simulink model "Sim_Riementrieb"  (R2019b)
settings: Solver=ode45  StartTime=0.0  StopTime=12  MaxStep=1e-3  RelTol=1e-7  AbsTol=1e-7  EnableMultiTasking=on
undefined symbols (not defined in the file or in its folder): parSys
libraries: cstblocks x2
settings Model: Creator=wke  LastModifiedBy=GF
settings SolverCC: AutoScaleAbsTol=off  ShapePreserveControl=EnableAll
settings DataIOCC: LimitDataPoints=on  SaveFormat=Array  SignalLoggingSaveFormat=ModelDataLogs  ReturnWorkspaceOutputs=off
settings OptimizationCC: ExpressionDepthLimit=2147483647  LifeSpan=inf
settings DebuggingCC: UnderspecifiedInitializationDetection=Classic  MergeDetectMultiDrivingBlocksExec=none  SolverPrmCheckMsg=warning  FcnCallInpInsideContextMsg=warning  StateNameClashWarn=warning  SFUnexpectedBacktrackingDiag=warning  SFNoUnconditionalDefaultTransitionDiag=warning  SFExecutionAtInitializationDiag=none  ArithmeticOperatorsInVariantConditions=warning
settings HardwareCC: ProdBitPerPointer=32  ProdBitPerSizeT=32  ProdBitPerPtrDiffT=32  ProdLargestAtomicFloat=None  ProdIntDivRoundTo=Undefined  ProdEndianess=Unspecified  ProdWordSize=32  ProdHWDeviceType=32-bit Generic
settings ModelReferenceCC: PropagateSignalLabelsOutOfModel=off
settings SFSimCC: SimUseLocalCustomCode=off  SimParseCustomCode=off  CustomCodeUndefinedFunction=UseInterfaceOnly
settings RTWCC: RTWUseLocalCustomCode=off
settings CodeAppCC: StateflowObjectComments=on
settings GRTTargetCC: TargetLangStandard=C89/C90 (ANSI)  GeneratePreprocessorConditionals=Disable all  CombineOutputUpdateFcns=off  GRTInterface=on
settings ConfigComp: CovMetricSettings=dw  CovHtmlReporting=on  CovSaveCumulativeToWorkspaceVar=on  CovSaveSingleToWorkspaceVar=on  CovExternalEMLEnable=off

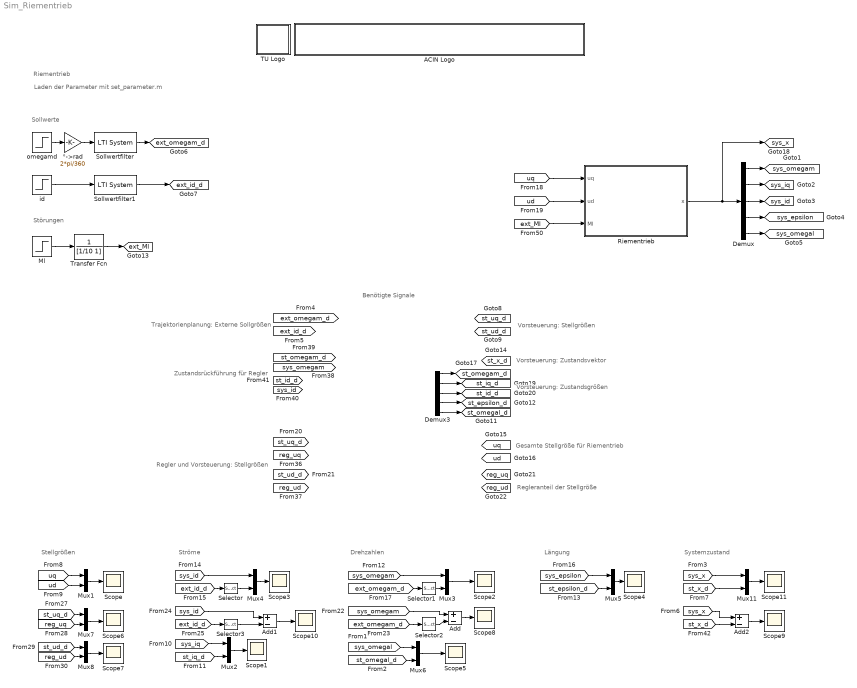
== system Sim_Riementrieb ==
  note: Regler und Vorsteuerung: Stellgrößen
  note: Zustandsrückführung für Regler
  note: Trajektorienplanung: Externe Sollgrößen
  note: Regleranteil der Stellgröße
  note: Gesamte Stellgröße für Riementrieb
  note: Vorsteuerung: Zustandsgrößen
  note: Vorsteuerung: Stellgrößen
  note: Riementrieb
  note: Laden der Parameter mit set_parameter.m
  note: Sollwerte
  note: Stellgrößen
  note: Ströme
  note: Drehzahlen
  note: Längung
  note: Störungen
  note: Systemzustand
  note: Benötigte Signale
  note: Vorsteuerung: Zustandsvektor
  ACIN Logo : Subsystem
      mask init:
      | s = get_param(gcb,'UserData');
      mask Display:
      | image(s.logo,[0 0 439 45]);
      | %axis image
  Add : Sum  Inputs=+-
  Add1 : Sum  Inputs=+-
  Add2 : Sum  Inputs=+-
  Demux : Demux  Outputs=5
  Demux3 : Demux  Outputs=5
  Ml : Step  Time=8  After=0.1  SampleTime=0
  Mux{1..8,11} (9 alike) : Mux  Inputs=2
  Riementrieb : Subsystem
  Scope{,1..11} (12 alike) : Scope
  Selector : Selector  InputPortWidth=2  IndexOptions=Index vector (dialog)  Indices=[1]  OutputSizes=1
  Selector1 : Selector  InputPortWidth=3  IndexOptions=Index vector (dialog)  Indices=[1]  OutputSizes=1
  Selector2 : Selector  InputPortWidth=3  IndexOptions=Index vector (dialog)  Indices=[1]  OutputSizes=1
  Selector3 : Selector  InputPortWidth=2  IndexOptions=Index vector (dialog)  Indices=[1]  OutputSizes=1
  Sollwertfilter : cstblocks/LTI System  sys=parReg.ssSF  IC=[]
  Sollwertfilter1 : cstblocks/LTI System  sys=parReg.ssSFi  IC=[]
  TU Logo : Subsystem
      mask init:
      | s = get_param(gcb,'UserData');
      mask Display: image(s.logo,[0 0 45 45]);
  Transfer Fcn : TransferFcn  Denominator=[1/10 1]
  id : Step  After=0.1  SampleTime=0
  omegamd : Step  Time=4  After=1000/60*360  SampleTime=0
  °->rad : Gain  Gain=2*pi/360
  tag scope: ext_Ml=global, ext_id_d=global, ext_omegam_d=global, reg_ud=global, reg_uq=global, st_epsilon_d=global, st_id_d=global, st_iq_d=global, st_omegal_d=global, st_omegam_d=global, st_ud_d=global, st_uq_d=global, st_x_d=global, sys_epsilon=global, sys_id=global, sys_iq=global, sys_omegal=global, sys_omegam=global, sys_x=global, ud=global, uq=global
  wires:
  °->rad/1 -> Sollwertfilter/1
  Sollwertfilter/1 -> [ext_omegam_d]
  Sollwertfilter1/1 -> [ext_id_d]
  id/1 -> Sollwertfilter1/1
  [uq] -> Mux1/1
  [ud] -> Mux1/2
  Mux1/1 -> Scope/1
  [sys_iq] -> Mux2/1
  [st_iq_d] -> Mux2/2
  Mux2/1 -> Scope1/1
  [sys_omegam] -> Mux3/1
  Mux3/1 -> Scope2/1
  [sys_id] -> Mux4/1
  [ext_id_d] -> Selector/1
  Mux4/1 -> Scope3/1
  [sys_epsilon] -> Mux5/1
  Mux5/1 -> Scope4/1
  [sys_omegal] -> Mux6/1
  Mux6/1 -> Scope5/1
  [ext_omegam_d] -> Selector1/1
  Selector1/1 -> Mux3/2
  Selector/1 -> Mux4/2
  [st_epsilon_d] -> Mux5/2
  [st_omegal_d] -> Mux6/2
  Add/1 -> Scope8/1
  [sys_omegam] -> Add/1
  [ext_omegam_d] -> Selector2/1
  Selector2/1 -> Add/2
  Add1/1 -> Scope10/1
  [sys_id] -> Add1/1
  [ext_id_d] -> Selector3/1
  Selector3/1 -> Add1/2
  Ml/1 -> Transfer Fcn/1
  omegamd/1 -> °->rad/1
  Transfer Fcn/1 -> [ext_Ml]
  [st_uq_d] -> Mux7/1
  [reg_uq] -> Mux7/2
  Mux7/1 -> Scope6/1
  [st_ud_d] -> Mux8/1
  [reg_ud] -> Mux8/2
  Mux8/1 -> Scope7/1
  Mux11/1 -> Scope11/1
  [sys_x] -> Mux11/1
  [st_x_d] -> Mux11/2
  Demux3/4 -> [st_epsilon_d]
  Demux3/5 -> [st_omegal_d]
  Demux3/1 -> [st_omegam_d]
  Demux3/2 -> [st_iq_d]
  Demux3/3 -> [st_id_d]
  Add2/1 -> Scope9/1
  [sys_x] -> Add2/1
  [st_x_d] -> Add2/2
  Demux/2 -> [sys_iq]
  Demux/1 -> [sys_omegam]
  Demux/3 -> [sys_id]
  Demux/4 -> [sys_epsilon]
  Demux/5 -> [sys_omegal]
  Riementrieb/1(x) -> [sys_x], Demux/1
  [uq] -> Riementrieb/1(uq)
  [ud] -> Riementrieb/2(ud)
  [ext_Ml] -> Riementrieb/3(Ml)
  ? -> [st_x_d], Demux3/1

== system Sim_Riementrieb/ACIN Logo ==

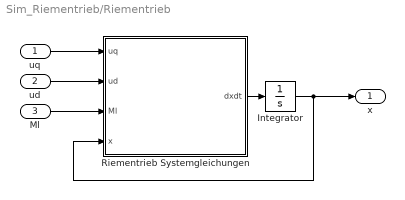
== system Sim_Riementrieb/Riementrieb ==
  uq : Inport
  ud : Inport  Port=2
  Ml : Inport  Port=3
  Integrator : Integrator  InitialCondition=parSys.x0
  Riementrieb Systemgleichungen : MATLAB Function  TreatAsAtomicUnit=on
  x : Outport  VectorParamsAs1DForOutWhenUnconnected=off
  wires:
  Ml/1 -> Riementrieb Systemgleichungen/3(Ml)
  ud/1 -> Riementrieb Systemgleichungen/2(ud)
  Integrator/1 -> x/1, Riementrieb Systemgleichungen/4(x)
  Riementrieb Systemgleichungen/1(dxdt) -> Integrator/1
  uq/1 -> Riementrieb Systemgleichungen/1(uq)

== system Sim_Riementrieb/TU Logo ==

== matlab function Sim_Riementrieb/Riementrieb/Riementrieb Systemgleichungen ==
  data: uq input; ud input; Ml input; x input; dxdt output; parSys parameter
function dxdt =fcn(uq,ud,Ml,x,parSys)
  dxdt=zeros(5,1);
  omegam=x(1);
  iq=x(2);
  id=x(3);
  epsilon=x(4);
  omegal=x(5);
  t3 = epsilon * epsilon;
  t6 = parSys.cr1 * epsilon + parSys.cr3 * t3 * epsilon;
  t10 = parSys.p * parSys.Phi;
  dt_omegam = 0.1e1 / parSys.Im * (0.2e1 * t6 * parSys.rm - parSys.dm * omegam + 0.3e1 / 0.2e1 * t10 * iq);
  t14 = 0.1e1 / parSys.Lm;
  t16 = parSys.Lm * parSys.p;
  dt_iq = 0.2e1 / 0.3e1 * t14 * (-parSys.Rm * iq + 0.3e1 / 0.2e1 * t16 * omegam * id - t10 * omegam + uq);
  dt_id = 0.2e1 / 0.3e1 * t14 * (-parSys.Rm * id - 0.3e1 / 0.2e1 * t16 * omegam * iq + ud);
  dt_epsilon = parSys.rl * omegal - parSys.rm * omegam;
  dt_omegal = 0.1e1 / parSys.Il * (-0.2e1 * t6 * parSys.rl - parSys.dl * omegal + Ml);
  dxdt=[dt_omegam;dt_iq;dt_id;dt_epsilon;dt_omegal];
end
